simulink subsystem "three_phases_generator"  (R2024b)
settings: Solver=VariableStepAuto  StartTime=0.0  StopTime=10.0  RelTol=1e-3
settings Model: Creator=antoinedaniel  LastModifiedBy=antoinedaniel

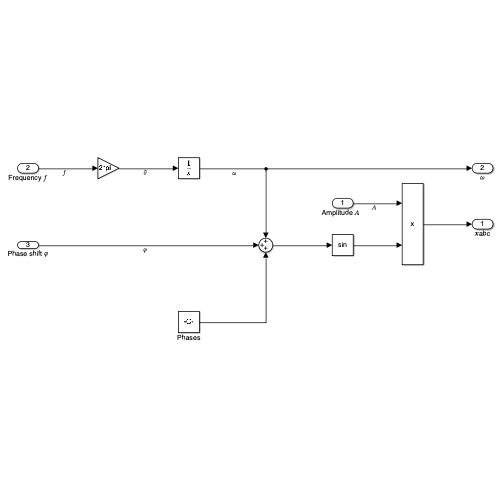
[thumbnail: Simulink's stored preview of the top-level diagram]
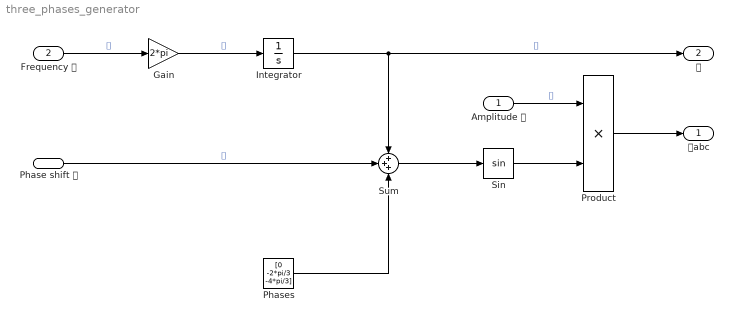
== system three_phases_generator ==
  "Amplitude 𝐴  " : Inport
  Frequency 𝑓 : Inport  Port=2
  Phase shift 𝜑 : Inport  Port=3
  Gain : Gain  Gain=2*pi
  Integrator : Integrator
  Phases : Constant  Value=[0 -2*pi/3 -4*pi/3]
  Product : Product
  Sin : Trigonometry
  Sum : Sum  Inputs=+++
  𝒙abc : Outport
  𝜔 : Outport  Port=2
  wires:
  Frequency 𝑓/1 -> Gain/1  "𝑓"
  Gain/1 -> Integrator/1  "𝜃"
  Phase shift 𝜑/1 -> Sum/2  "𝜑"
  Integrator/1 -> Sum/1, 𝜔/1  "𝜔"
  Sum/1 -> Sin/1
  "Amplitude 𝐴  "/1 -> Product/1  "𝐴"
  Sin/1 -> Product/2
  Product/1 -> 𝒙abc/1
  Phases/1 -> Sum/3
